simulink model "IM_VF_PWM"  (R2014a)
settings: Solver=ode23tb  StartTime=0.0  StopTime=1  RelTol=1e-3
libraries: powerlib x7, powerlib_meascontrol x3, simulink x1
settings Model: Creator=ninad gaikawad  LastModifiedBy=ninad gaikawad

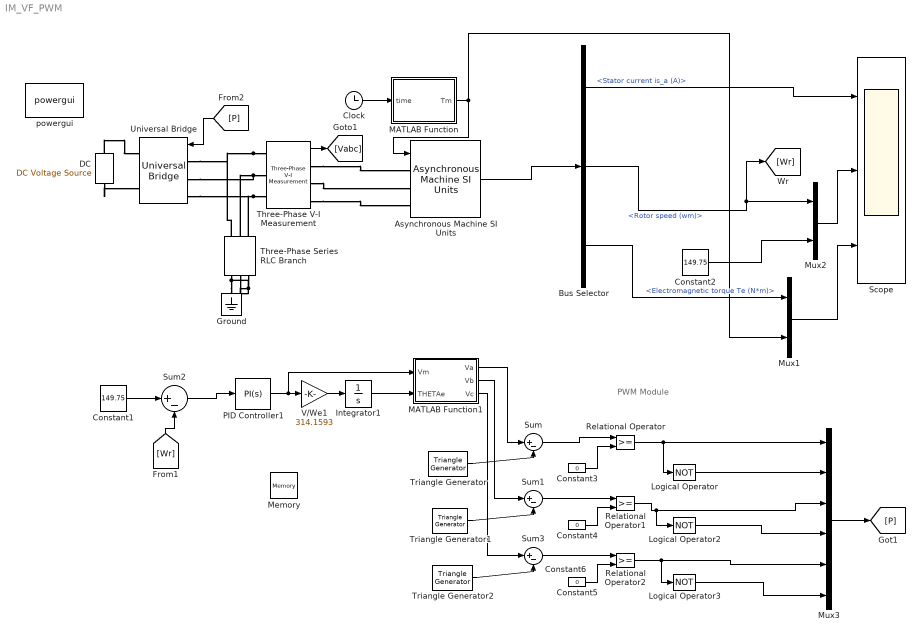
== system IM_VF_PWM ==
  note: PWM Module
  Asynchronous Machine SI Units : powerlib/Machines/Asynchronous Machine SI Units  PresetModel="15:  5.4 HP (4KW)   400 V  50Hz 1430 RPM"  MechanicalLoad=Torque Tm  ShowDetailedParameters=on  RotorType=Squirrel-cage  ReferenceFrame=Rotor  Units=SI  MeasurementBus=off  NominalParameters=[4000 400 50]  Stator=[1.405 0.005839]  Rotor=[1.395 0.005839]  Cage1=[ 0.022 0.226/377]  Cage2=[ 0.022 0.226/377]  Lm=0.1722  Mechanical=[0.0131 0.002985 2]  PolePairs=2  InitialConditions=[1 0 0 0 0 0 0 0]  SimulateSaturation=off  Saturation=[14.03593122, 27.81365428, 53.79336849, 72.68890987, 97.98006896, 148.6815601, 215.7428561, 302.9841135, 420.4778367 ; 230, 322, 414, 460, 506, 552, 598, 644, 690]  LoadFlowParameters=1492000  TsPowergui=0  TsBlock=-1  IterativeModel=Trapezoidal non iterative  Pmec=0
  Bus Selector : BusSelector  OutputSignals=Stator measurements.Stator current is_a (A),Mechanical.Rotor speed (wm),Mechanical.Electromagnetic torque Te (N*m)
  Clock : Clock
  Constant1 : Constant  Value=149.75
  Constant2 : Constant  Value=149.75
  Constant{3..6} (4 alike) : Constant  Value=0
  "DC " : powerlib/Electrical Sources/DC Voltage Source  Amplitude=565.7  Measurements=None
  Ground : powerlib/Elements/Ground  LConnTagsString=a
  Integrator1 : Integrator
  Logical Operator : Logic  Operator=NOT  AllPortsSameDT=off  OutDataTypeStr=boolean
  Logical Operator2 : Logic  Operator=NOT  AllPortsSameDT=off  OutDataTypeStr=boolean
  Logical Operator3 : Logic  Operator=NOT  AllPortsSameDT=off  OutDataTypeStr=boolean
  MATLAB Function : MATLAB Function  TreatAsAtomicUnit=on
  MATLAB Function1 : MATLAB Function  TreatAsAtomicUnit=on
  Memory : Memory
  Mux1 : Mux  Inputs=2
  Mux2 : Mux  Inputs=2
  Mux3 : Mux  Inputs=6
  PID Controller1 : simulink/Continuous/PID Controller  Controller=PI  TimeDomain=Continuous-time  SampleTime=1  IntegratorMethod=Forward Euler  FilterMethod=Forward Euler  Form=Parallel  P=2.5e-2  I=2.5e-1  D=0  N=100  InitialConditionSource=internal  InitialConditionForIntegrator=0  InitialConditionForFilter=0  ExternalReset=none  LimitOutput=on  UpperSaturationLimit=0.99  LowerSaturationLimit=0  LinearizeAsGain=on  AntiWindupMode=clamping  Kb=1  TrackingMode=off  Kt=1  PParamMin=[]  PParamMax=[]  IParamMin=[]  IParamMax=[]  DParamMin=[]  DParamMax=[]  NParamMin=[]  NParamMax=[]  KbParamMin=[]  KbParamMax=[]  KtParamMin=[]  KtParamMax=[]  POutMin=[]  POutMax=[]  IOutMin=[]  IOutMax=[]  DOutMin=[]  DOutMax=[]  NOutMin=[]  NOutMax=[]  KbOutMin=[]  KbOutMax=[]  KtOutMin=[]  KtOutMax=[]  IntegratorOutMin=[]  IntegratorOutMax=[]  FilterOutMin=[]  FilterOutMax=[]  SumOutMin=[]  SumOutMax=[]  SumI1OutMin=[]  SumI1OutMax=[]  SumI2OutMin=[]  SumI2OutMax=[]  SumI3OutMin=[]  SumI3OutMax=[]  SumDOutMin=[]  SumDOutMax=[]  SaturationOutMin=[]  SaturationOutMax=[]  IntegratorContinuousStateAttributes=''  IntegratorStateMustResolveToSignalObject=off  IntegratorRTWStateStorageClass=Auto  FilterContinuousStateAttributes=''  FilterStateMustResolveToSignalObject=off  FilterRTWStateStorageClass=Auto
  Relational Operator : RelationalOperator  OutDataTypeStr=boolean
  Relational Operator1 : RelationalOperator  OutDataTypeStr=boolean
  Relational Operator2 : RelationalOperator  OutDataTypeStr=boolean
  Scope : Scope  NumInputPorts=3
      settings: YMin=-5~-5~-5  YMax=5~5~5
  Sum{,1..3} (4 alike) : Sum  Inputs=|+-
  Three-Phase Series RLC Branch : powerlib/Elements/Three-Phase Series RLC Branch  LConnTagsString=A|B|C  RConnTagsString=A|B|C  BranchType=R  Resistance=1e6  Inductance=1e-3  Capacitance=1e-6  Measurements=None
  Three-Phase V-I Measurement : powerlib/Measurements/Three-Phase V-I Measurement  VoltageMeasurement=phase-to-phase  SetLabelV=off  LabelV=Vabc  Vpu=off  VpuLL=off  CurrentMeasurement=no  SetLabelI=off  LabelI=Iabc  Ipu=off  Pbase=100e6  Vbase=500e3  OutputType=Complex  PhasorSimulation=off  PSBequivalent=0
  Triangle Generator : powerlib_meascontrol/Pulse & Signal Generators/Triangle Generator  Freq=1e3  Phase=0  Ts=0
  Triangle Generator1 : powerlib_meascontrol/Pulse & Signal Generators/Triangle Generator  Freq=1e3  Phase=-120  Ts=0
  Triangle Generator2 : powerlib_meascontrol/Pulse & Signal Generators/Triangle Generator  Freq=1e3  Phase=-240  Ts=0
  Universal Bridge : powerlib/Power Electronics/Universal Bridge  Arms=3  SnubberResistance=1e5  SnubberCapacitance=inf  Device=IGBT / Diodes  Ron=1e-3  Lon=0  ForwardVoltages="[  0  0  ]"  ForwardVoltage=0  GTOparameters=[ 10e-6 , 20e-6 ]  IGBTparameters=[ 1e-6 , 2e-6 ]  Measurements=None  Measurements_2=None  converterType=Rectifier
  V/We1 : Gain  Gain=314.1593
  powergui : powerlib/powergui  Priority=1  SimulationMode=Continuous  SolverType=Tustin  SampleTime=50e-6  frequency=60  SPID=off  DisableSnubberDevices=off  DisableRonSwitches=off  DisableVfSwitches=off  SwTol=0  Interpol=off  DisplayEquations=off  Ts=0  methode=off  frequencyindice=50  Pbase=100e6  ErrMax=1e-4  Iterations=50  UnitsV=kV  UnitsW=MW  FunctionMessages=off  echomessages=off  HookPort=off  EnableUseOfTLC=off  x0status=blocks  RestoreLinks=warning  ResistiveCurrentMeasurement=off  Frange=[0:2:500]  Ylog=off  Xlog=on  ShowGrid=off  save=off  variable=ZData  structure=0  ZoomFFT=off  StartTime=0.0  cycles=1  DisplayStyle=1  fundamental=60  FreqAxis=off  MaxFrequency=1000  frequencyindicesteady=1  RmsSteady=1  display=off
  wires:
  Asynchronous Machine SI Units/1 -> Bus Selector/1
  Mux1/1 -> Scope/3
  Mux2/1 -> Scope/2
  [P] -> Universal Bridge/1
  Three-Phase V-I Measurement/1 -> [Vabc]
  Bus Selector/1 -> Scope/1  "<Stator current is_a (A)>"
  Bus Selector/2 -> Mux2/1, [Wr]  "<Rotor speed (wm)>"
  Bus Selector/3 -> Mux1/1  "<Electromagnetic torque Te (N*m)>"
  Constant2/1 -> Mux2/2
  Constant1/1 -> Sum2/1
  V/We1/1 -> Integrator1/1
  Integrator1/1 -> MATLAB Function1/2(THETAe)
  PID Controller1/1 -> MATLAB Function1/1(Vm), V/We1/1
  Clock/1 -> MATLAB Function/1(time)
  MATLAB Function/1(Tm) -> Asynchronous Machine SI Units/1, Mux1/2
  [Wr] -> Sum2/2
  Sum2/1 -> PID Controller1/1
  Triangle Generator/1 -> Sum/2
  Triangle Generator1/1 -> Sum1/2
  Triangle Generator2/1 -> Sum3/2
  MATLAB Function1/1(Va) -> Sum/1
  MATLAB Function1/2(Vb) -> Sum1/1
  MATLAB Function1/3(Vc) -> Sum3/1
  Sum/1 -> Relational Operator/1
  Constant3/1 -> Relational Operator/2
  Constant4/1 -> Relational Operator1/2
  Sum1/1 -> Relational Operator1/1
  Sum3/1 -> Relational Operator2/1
  Constant6/1 -> Relational Operator2/2
  Relational Operator/1 -> Logical Operator/1, Mux3/1
  Relational Operator1/1 -> Logical Operator2/1, Mux3/3
  Logical Operator2/1 -> Mux3/4
  Logical Operator/1 -> Mux3/2
  Relational Operator2/1 -> Logical Operator3/1, Mux3/5
  Logical Operator3/1 -> Mux3/6
  Mux3/1 -> [P]
  connections:
  Three-Phase V-I Measurement/LConn2 -- Universal Bridge/LConn2 -- Three-Phase Series RLC Branch/LConn2
  Three-Phase V-I Measurement/LConn1 -- Universal Bridge/LConn1 -- Three-Phase Series RLC Branch/LConn1
  Three-Phase V-I Measurement/LConn3 -- Universal Bridge/LConn3 -- Three-Phase Series RLC Branch/LConn3
  Ground/LConn1 -- Three-Phase Series RLC Branch/RConn3 -- Three-Phase Series RLC Branch/RConn1 -- Three-Phase Series RLC Branch/RConn2
  Three-Phase V-I Measurement/RConn2 -- Asynchronous Machine SI Units/LConn2
  "DC "/RConn1 -- Universal Bridge/RConn1
  Three-Phase V-I Measurement/RConn3 -- Asynchronous Machine SI Units/LConn3
  "DC "/LConn1 -- Universal Bridge/RConn2
  Three-Phase V-I Measurement/RConn1 -- Asynchronous Machine SI Units/LConn1

== matlab function IM_VF_PWM/MATLAB Function1 ==
  settings: updateMethod=CONTINUOUS
  data: Vm input; Va output; THETAe input; Vb output; Vc output
function [Va,Vb,Vc] = fcnn(Vm,THETAe)
 Va=Vm*sin(THETAe);
 Vb=Vm*sin(THETAe-(2*pi/3));
 Vc=Vm*sin(THETAe+(2*pi/3));

== matlab function IM_VF_PWM/MATLAB Function ==
  data: Tm output; time input
function Tm = mechanical_torque(time)

if (time < 0.4 || time > 0.6)
Tm = 0;
else
Tm = 26.71;
end
end
